simulink model "lab04part20"  (R2015a)
settings: Solver=ode45  StartTime=0.0  StopTime=50.0  RelTol=1e-3
settings Model: Creator=dg  LastModifiedBy=dg

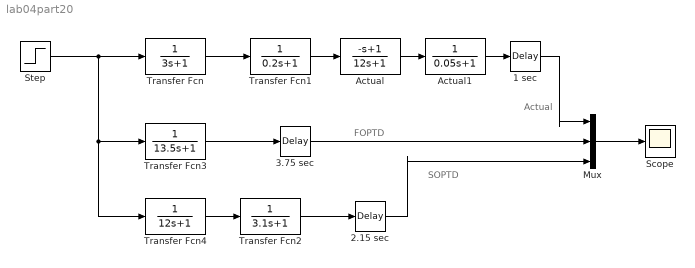
== system lab04part20 ==
  note: Actual
  note: SOPTD
  note: FOPTD
  1 sec : TransportDelay
  "2.15 sec " : TransportDelay  DelayTime=2.15
  "3.75 sec " : TransportDelay  DelayTime=3.75
  Actual : TransferFcn  Numerator=[-1 1]  Denominator=[12 1]
  Actual1 : TransferFcn  Denominator=[0.05 1]
  Mux : Mux  Inputs=3
  Scope : Scope
      settings: ShowLegends=on
  Step : Step  SampleTime=0
  Transfer Fcn : TransferFcn  Denominator=[3 1]
  Transfer Fcn1 : TransferFcn  Denominator=[0.2 1]
  Transfer Fcn2 : TransferFcn  Denominator=[3.1 1]
  Transfer Fcn3 : TransferFcn  Denominator=[13.5 1]
  Transfer Fcn4 : TransferFcn  Denominator=[12 1]
  wires:
  Step/1 -> Transfer Fcn4/1, Transfer Fcn3/1, Transfer Fcn/1
  Transfer Fcn/1 -> Transfer Fcn1/1
  Transfer Fcn1/1 -> Actual/1
  Mux/1 -> Scope/1
  Actual/1 -> Actual1/1
  Transfer Fcn3/1 -> "3.75 sec "/1
  Transfer Fcn4/1 -> Transfer Fcn2/1
  "3.75 sec "/1 -> Mux/2
  "2.15 sec "/1 -> Mux/3
  Transfer Fcn2/1 -> "2.15 sec "/1
  Actual1/1 -> 1 sec/1
  1 sec/1 -> Mux/1
